simulink model "exp3_partial_shading (1)"  (R2023a)
settings: Solver=ode23tb  StartTime=0.0  StopTime=10  MaxStep=3e-3  RelTol=1e-3
libraries: spsDiodeLib x4, spsPVArrayLib x4, spspowerguiLib x2, spsCurrentMeasurementLib x1, simulink x1, spsControlledCurrentSourceLib x1, spsVoltageMeasurementLib x1
settings Model: Creator=ayyrao  LastModifiedBy=astit
settings SolverCC: AlgebraicLoopSolver=TrustRegion
settings DataIOCC: ReturnWorkspaceOutputs=off
settings DebuggingCC: UnconnectedInputMsg=warning  UnconnectedOutputMsg=warning  UnconnectedLineMsg=warning  ArithmeticOperatorsInVariantConditions=warning
settings ModelReferenceCC: EnableRefExpFcnMdlSchedulingChecks=on
settings SFSimCC: SimUseLocalCustomCode=off  CustomCodeUndefinedFunction=UseInterfaceOnly
settings RTWCC: RTWUseLocalCustomCode=off  DLArmComputeVersion=19.05

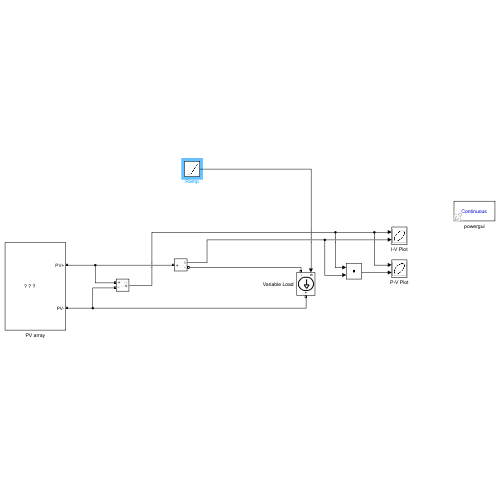
[thumbnail: Simulink's stored preview of the top-level diagram]
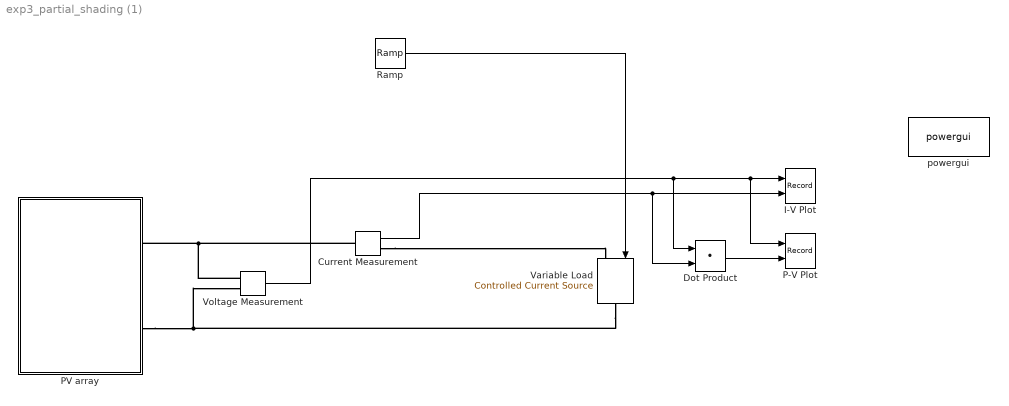
== system exp3_partial_shading (1) ==
  Current Measurement : spsCurrentMeasurementLib/Current Measurement  PhasorSimulation=off  OutputType=Complex  PSBequivalent=0
  Dot Product : DotProduct  OutDataTypeStr=Inherit: Inherit via internal rule
  I-V Plot : Record  FileSettingsInternal="{\"entries\":[{\"content\":{\"excelSettings\":{\"content\":{},\"type\":\"Streamout.ExcelSettings\"}},\"type\":\"Streamout.FileSettingStorage\",\"uuid\":\"\"}],\"packageUris\":[\"http:\\/\\/schema.mathworks.com\\/mf0\\/streamout_blocks\\/R2020a\"],\"version\":\"1.0\"}"  Layout=[1 1]  SignalsInternal="{\"entries\":[{\"content\":{\"signals\":[{\"content\":{\"blockPath\":[],\"dimensions\":[1],\"domain\":\"\",\"lineColor\":\"#a2142f\",\"plots\":[1],\"port\":1,\"sid\":[\"\"],\"signalID\":63,\"signalName\":\"Voltage Measurement\"},\"type\":\"RecordBlkView.Signal\",\"uuid\":\"\"},{\"content\":{\"blockPath\":[],\"dimensions\":[1],\"domain\":\"\",\"lineColor\":\"#139fff\",\"plots\":[1],\"port\":2,\"sid\":[\"\"],\"signalID\":67,\"signalName\":\"Current Measurement\"},\"type\":\"RecordBlkView.Signal\",\"uuid\":\"\"}]},\"type\":\"RecordBlkView.InputSignals\",\"uuid\":\"\"}],\"packageUris\":[\"http:\\/\\/schema.mathworks.com\\/mf0\\/streamout_blocks\\/R2020a\"],\"version\":\"1.0\"}"  VisualizationBindings="{\"xyplotplugin\":{\"info\":[{\"series\":[{\"bindingParametersList\":[{\"parameter\":\"X-Axis\",\"signalID\":63,\"signalName\":\"Voltage Measurement\"},{\"parameter\":\"Y-Axis\",\"signalID\":67,\"signalName\":\"Current Measurement\"}],\"seriesID\":5876}],\"subplotID\":1}]}}"  CompatibilityTag=XY  st=-1
  P-V Plot : Record  FileSettingsInternal="{\"entries\":[{\"content\":{\"excelSettings\":{\"content\":{},\"type\":\"Streamout.ExcelSettings\"}},\"type\":\"Streamout.FileSettingStorage\",\"uuid\":\"\"}],\"packageUris\":[\"http:\\/\\/schema.mathworks.com\\/mf0\\/streamout_blocks\\/R2020a\"],\"version\":\"1.0\"}"  Layout=[1 1]  SignalsInternal="{\"entries\":[{\"content\":{\"signals\":[{\"content\":{\"blockPath\":[],\"dimensions\":[1],\"domain\":\"\",\"lineColor\":\"#a2142f\",\"plots\":[1],\"port\":1,\"sid\":[\"\"],\"signalID\":71,\"signalName\":\"Voltage Measurement\"},\"type\":\"RecordBlkView.Signal\",\"uuid\":\"\"},{\"content\":{\"blockPath\":[],\"dimensions\":[1],\"domain\":\"\",\"lineColor\":\"#139fff\",\"plots\":[1],\"port\":2,\"sid\":[\"\"],\"signalID\":75,\"signalName\":\"Dot Product\"},\"type\":\"RecordBlkView.Signal\",\"uuid\":\"\"}]},\"type\":\"RecordBlkView.InputSignals\",\"uuid\":\"\"}],\"packageUris\":[\"http:\\/\\/schema.mathworks.com\\/mf0\\/streamout_blocks\\/R2020a\"],\"version\":\"1.0\"}"  VisualizationBindings="{\"xyplotplugin\":{\"info\":[{\"series\":[{\"bindingParametersList\":[{\"parameter\":\"X-Axis\",\"signalID\":71,\"signalName\":\"Voltage Measurement\"},{\"parameter\":\"Y-Axis\",\"signalID\":75,\"signalName\":\"Dot Product\"}],\"seriesID\":34104}],\"subplotID\":1}]}}"  CompatibilityTag=XY  st=-1
  PV array : Subsystem
      mask Display: image('E:\mathworks-up\mppt\2x2-PV-array-with-bypass-diodes-across-each-PV-module-and-blocking-diodes-a-in-the-top.png');
  Ramp : simulink/Sources/Ramp  slope=1  start=0  InitialOutput=0
  Variable Load : spsControlledCurrentSourceLib/Controlled Current Source  Initialize=on  Source_Type=AC  Amplitude=0  Phase=0  Frequency=0  Measurements=None
  Voltage Measurement : spsVoltageMeasurementLib/Voltage Measurement  PhasorSimulation=off  OutputType=Complex  PSBequivalent=0
  powergui : spspowerguiLib/powergui  Priority=1  SimulationMode=Continuous  SampleTime=50e-6  frequency=60  Iterations=50  frequencyindice=0  Pbase=100e6  ErrMax=1e-4  UnitsV=kV  UnitsW=MW  buscounter=0  FunctionMessages=off  echomessages=off  EnableUseOfTLC=off  CurrentSourceSwitches=off  DisableSnubberDevices=off  DisableRonSwitches=off  DisableVfSwitches=off  DisplayEquations=off  AutomaticDiscreteSolvers=off  SolverType=Tustin/Backward Euler (TBE)  Interpol=off  ExternalGateDelay=off  methode=off  Ts=100  x0status=blocks  SPID=on  SwTol=0  HookPort=off  NonlinearTolerance=1e-4  nMaxIteration=100  ContinueOnMaxIteration=off  RestoreLinks=warning  ResistiveCurrentMeasurement=off  Frange=[0:2:500]  Ylog=off  Xlog=on  ShowGrid=off  save=off  variable=ZData  structure=0  ZoomFFT=off  StartTime=0.0  cycles=1  DisplayStyle=1  fundamental=60  FreqAxis=off  MaxFrequency=1000  frequencyindicesteady=1  RmsSteady=1  display=off
  wires:
  Ramp/1 -> Variable Load/1
  Current Measurement/1 -> Dot Product/2, I-V Plot/2
  Voltage Measurement/1 -> Dot Product/1, P-V Plot/1, I-V Plot/1
  Dot Product/1 -> P-V Plot/2
  connections:
  Voltage Measurement/LConn1 -- Current Measurement/LConn1 -- PV array/RConn1
  PV array/RConn2 -- Variable Load/RConn1 -- Voltage Measurement/LConn2
  Current Measurement/RConn1 -- Variable Load/LConn1

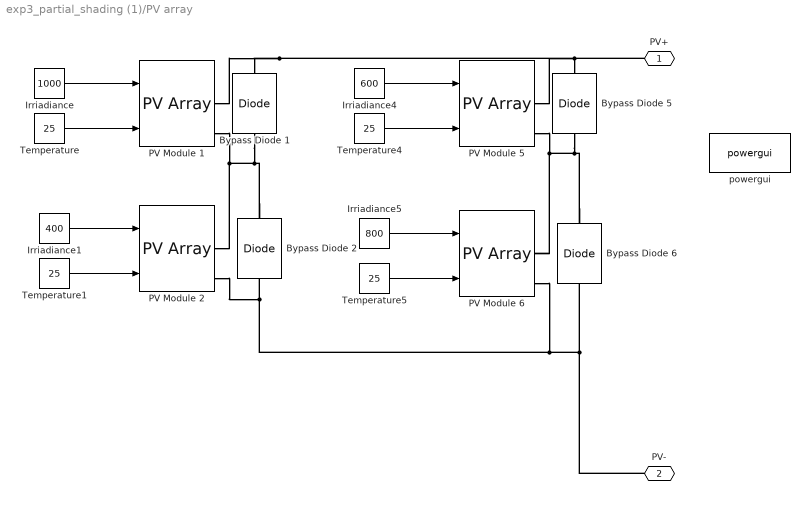
== system exp3_partial_shading (1)/PV array ==
  Bypass Diode {1..2,5..6} (4 alike) : spsDiodeLib/Diode  Ron=0.001  Lon=0  Vf=0.8  IC=0  UseSnubber=off  Rs=500  Cs=250e-9  Measurements=off
  Irriadiance : Constant  Value=1000
  Irriadiance1 : Constant  Value=400
  Irriadiance4 : Constant  Value=600
  Irriadiance5 : Constant  Value=800
  PV Module 1 : spsPVArrayLib/PV Array  Npar=1  Nser=1  PlotType=array @ 25 deg.C & specified irradiances  S_vec="[ 1000 800  600 400 200 ]"  Temp_C_vec="[ 45 25  ]"  ModuleName=User-defined  PlotWhenSelected=off  Pm=59.85  Ncell=36  Voc=21.1  Isc=3.8  Vm=17.1  Im=3.5  beta_Voc_pc=-0.8  alpha_Isc_pc=0.00247  beta_Voc=-0.1688  alpha_Isc=9.386e-05  IL=3.8366  I0=1.3941e-06  nI=1.5406  Rsh=283.3724  Rs=0.10363  RobustModel=off  RobustCellTemperature=313.3991  BAL=off  Tc=1e-6  Tfilter=5e-5
  PV Module 2 : spsPVArrayLib/PV Array  Npar=1  Nser=1  PlotType=array @ 1000 W/m2 & specified temperatures  S_vec="[ 1000  500  100 ]"  Temp_C_vec="[ 45 25  ]"  ModuleName=User-defined  PlotWhenSelected=off  Pm=59.85  Ncell=36  Voc=21.1  Isc=3.8  Vm=17.1  Im=3.5  beta_Voc_pc=-0.8  alpha_Isc_pc=0.00247  beta_Voc=-0.1688  alpha_Isc=9.386e-05  IL=3.8366  I0=1.3941e-06  nI=1.5406  Rsh=283.3724  Rs=0.10363  RobustModel=off  RobustCellTemperature=313.3991  BAL=off  Tc=1e-6  Tfilter=5e-5
  PV Module 5 : spsPVArrayLib/PV Array  Npar=1  Nser=1  PlotType=array @ 25 deg.C & specified irradiances  S_vec="[ 1000 800  600 400 200 ]"  Temp_C_vec="[ 45 25  ]"  ModuleName=User-defined  PlotWhenSelected=off  Pm=59.85  Ncell=36  Voc=21.1  Isc=3.8  Vm=17.1  Im=3.5  beta_Voc_pc=-0.8  alpha_Isc_pc=0.00247  beta_Voc=-0.1688  alpha_Isc=9.386e-05  IL=3.8366  I0=1.3941e-06  nI=1.5406  Rsh=283.3724  Rs=0.10363  RobustModel=off  RobustCellTemperature=313.3991  BAL=off  Tc=1e-6  Tfilter=5e-5
  PV Module 6 : spsPVArrayLib/PV Array  Npar=1  Nser=1  PlotType=array @ 1000 W/m2 & specified temperatures  S_vec="[ 1000  500  100 ]"  Temp_C_vec="[ 45 25  ]"  ModuleName=User-defined  PlotWhenSelected=off  Pm=59.85  Ncell=36  Voc=21.1  Isc=3.8  Vm=17.1  Im=3.5  beta_Voc_pc=-0.8  alpha_Isc_pc=0.00247  beta_Voc=-0.1688  alpha_Isc=9.386e-05  IL=3.8366  I0=1.3941e-06  nI=1.5406  Rsh=283.3724  Rs=0.10363  RobustModel=off  RobustCellTemperature=313.3991  BAL=off  Tc=1e-6  Tfilter=5e-5
  Temperature{,1,4..5} (4 alike) : Constant  Value=25
  powergui : spspowerguiLib/powergui  Priority=1  SimulationMode=Continuous  SampleTime=50e-6  frequency=60  Iterations=50  frequencyindice=0  Pbase=100e6  ErrMax=1e-4  UnitsV=kV  UnitsW=MW  buscounter=0  FunctionMessages=off  echomessages=off  EnableUseOfTLC=off  CurrentSourceSwitches=off  DisableSnubberDevices=off  DisableRonSwitches=off  DisableVfSwitches=off  DisplayEquations=off  AutomaticDiscreteSolvers=off  SolverType=Tustin/Backward Euler (TBE)  Interpol=off  ExternalGateDelay=off  methode=off  Ts=100  x0status=blocks  SPID=on  SwTol=0  HookPort=off  NonlinearTolerance=1e-4  nMaxIteration=100  ContinueOnMaxIteration=off  RestoreLinks=warning  ResistiveCurrentMeasurement=off  Frange=[0:2:500]  Ylog=off  Xlog=on  ShowGrid=off  save=off  variable=ZData  structure=0  ZoomFFT=off  StartTime=0.0  cycles=1  DisplayStyle=1  fundamental=60  FreqAxis=off  MaxFrequency=1000  frequencyindicesteady=1  RmsSteady=1  display=off
  PV+ : PMIOPort  Side=Right
  PV- : PMIOPort  Port=2  Side=Right
  wires:
  Temperature/1 -> PV Module 1/2
  Temperature1/1 -> PV Module 2/2
  Irriadiance/1 -> PV Module 1/1
  Irriadiance1/1 -> PV Module 2/1
  Irriadiance5/1 -> PV Module 6/1
  Temperature5/1 -> PV Module 6/2
  Irriadiance4/1 -> PV Module 5/1
  Temperature4/1 -> PV Module 5/2
  connections:
  Bypass Diode 2/RConn1 -- Bypass Diode 1/LConn1 -- PV Module 1/RConn2 -- PV Module 2/RConn1
  Bypass Diode 5/RConn1 -- PV+/RConn1 -- PV Module 5/RConn1 -- PV Module 1/RConn1 -- Bypass Diode 1/RConn1
  PV-/RConn1 -- Bypass Diode 2/LConn1 -- PV Module 2/RConn2 -- PV Module 6/RConn2 -- Bypass Diode 6/LConn1
  Bypass Diode 6/RConn1 -- Bypass Diode 5/LConn1 -- PV Module 6/RConn1 -- PV Module 5/RConn2
